simulink model "TAYCAN_MODEL"  (R2025b)
settings: Solver=ode23t  StartTime=0.0  StopTime=10000  RelTol=1e-3
values from neighbouring files (symbols this model uses):
  g = 9.81    [DRIVE_CYCLE_GEN.m]    (also in TAYCAN_PARAM_LOAD.m)
  L = 500    [TAYCAN_PARAM_LOAD.m]
  Max_brake_pressure_F_Bar = 200e5    (= 20000000)    [TAYCAN_PARAM_LOAD.m]
  Max_brake_pressure_R_Bar = 200e5    (= 20000000)    [TAYCAN_PARAM_LOAD.m]
  Max_torque_curve_F_Nm = Torque_x * Max_torque_curve_F_set    [Model_Sweeper.m]    (also in TAYCAN_PARAM_LOAD.m = [340;340;340;340;340;340;288.55;247.42;216.63;192.44;173.11;)
  Max_torque_curve_R_Nm = Torque_x * Max_torque_curve_R_set    [Model_Sweeper.m]    (also in TAYCAN_PARAM_LOAD.m = [900.00;900.00;900.00;900.00;900.00;900.00;900.00;898.90;785)
  Max_torque_generator_Nm = -350    [TAYCAN_PARAM_LOAD.m]
  Np = ceil(Ipack / Imax)    [Model_Sweeper.m]    (also in TAYCAN_PARAM_LOAD.m = 33)
  Ns = 198    [TAYCAN_PARAM_LOAD.m]
  regen_bias = 0.3    [TAYCAN_PARAM_LOAD.m]
  RPM_curve_RPM_F = (0:1000:RPM_max_RPM_F)'    [TAYCAN_PARAM_LOAD.m]
  RPM_curve_RPM_R = (0:1000:RPM_max_RPM_R)'    [TAYCAN_PARAM_LOAD.m]
  shift_down_v = shift_down_v_set(ids)    [Model_Sweeper.m]    (also in TAYCAN_PARAM_LOAD.m = 60)
  shift_up_v = shift_up_v_set(ids)    [Model_Sweeper.m]    (also in TAYCAN_PARAM_LOAD.m = 80)
  Tot_vehicle_mass_kg = Vehicle_mass_unladen_kg + Driver_mass_kg + batt_mass    [Model_Sweeper.m]    (also in TAYCAN_PARAM_LOAD.m = 2462.38)
  V_init = 4.2    [TAYCAN_PARAM_LOAD.m]
  VelDist = struct()    [DRIVE_CYCLE_GEN.m]    (also in VelocityVsDistance.mat = )
undefined symbols (not defined in the file or in its folder): Driver_Ki, Driver_Kp, Max_torque_motor_F__Nm, Max_torque_motor_R__Nm, Neg, Pos
libraries: fl_lib x23, nesl_utility x16, sdl_lib x15, batteryecm_lib x1, autolibshared x1
(part 2 of 2)

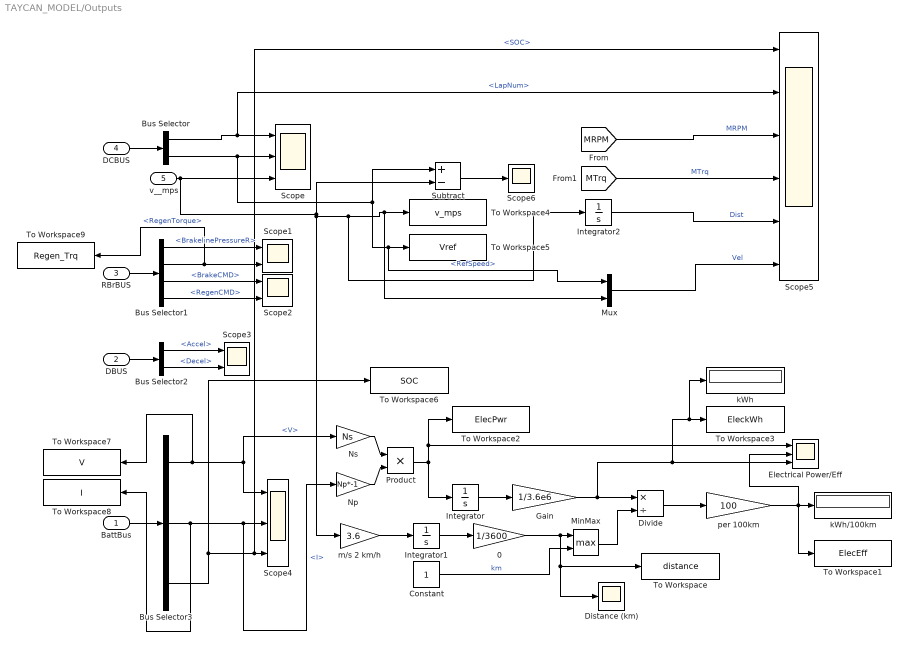
== system TAYCAN_MODEL/Outputs ==
  BattBus : Inport
  DBUS : Inport  Port=2
  RBrBUS : Inport  Port=3
  DCBUS : Inport  Port=4
  v__mps : Inport  Port=5
  0 : Gain  Gain=1/3600
  Bus Selector : BusSelector  OutputSignals=LapNum,RefSpeed
  Bus Selector1 : BusSelector  OutputSignals=BrakelinePressureR,RegenTorque,BrakeCMD,RegenCMD
  Bus Selector2 : BusSelector  OutputSignals=Info.Accel,Info.Decel
  Bus Selector3 : BusSelector  OutputSignals=V,I,SOC
  Constant : Constant
  Distance (km) : Scope
      settings: DataLoggingVariableName=ScopeData8
  Divide : Product  Inputs=*/
  Electrical Power/Eff : Scope  NumInputPorts=3
      settings: DataLoggingVariableName=ScopeData7
  Gain : Gain  Gain=1/3.6e6
  Integrator : Integrator
  Integrator1 : Integrator
  Integrator2 : Integrator
  MinMax : MinMax  Function=max  Inputs=2
  Mux : Mux  Inputs=2
  Np : Gain  Gain=Np*-1
  Ns : Gain  Gain=Ns
  Product : Product
  Scope : Scope  NumInputPorts=3
      settings: ActiveDisplayYMinimum=-0.24999999999999994  ActiveDisplayYMaximum=2.25
  Scope1 : Scope  NumInputPorts=2
      settings: ActiveDisplayYMinimum=-2.4999999999999995E+6  ActiveDisplayYMaximum=2.25E+7
  Scope2 : Scope  NumInputPorts=2
      settings: ActiveDisplayYMinimum=-0.087499999999999981  ActiveDisplayYMaximum=0.7875  DataLoggingVariableName=ScopeData2
  Scope3 : Scope  NumInputPorts=2
      settings: ActiveDisplayYMinimum=-0.12499999999999997  ActiveDisplayYMaximum=1.125  DataLoggingVariableName=ScopeData3
  Scope4 : Scope  NumInputPorts=3
      settings: ActiveDisplayYMinimum=1.4182763065735668  ActiveDisplayYMaximum=4.8626794045097581  DataLoggingVariableName=ScopeData4
  Scope5 : Scope  NumInputPorts=6
      settings: ActiveDisplayYMinimum=0.63060484486680279  ActiveDisplayYMaximum=0.81648445711282258  DataLoggingVariableName=ScopeData6
  Scope6 : Scope
      settings: ActiveDisplayYMinimum=-58.874697621468819  ActiveDisplayYMaximum=25.807756510642971  DataLoggingVariableName=ScopeData9
  Subtract : Sum  Inputs=+-
  To Workspace : ToWorkspace  VariableName=distance  SaveFormat=Timeseries  SampleTime=-1
  To Workspace1 : ToWorkspace  VariableName=ElecEff  SaveFormat=Timeseries  SampleTime=-1
  To Workspace2 : ToWorkspace  VariableName=ElecPwr  SaveFormat=Timeseries  SampleTime=-1
  To Workspace3 : ToWorkspace  VariableName=EleckWh  SaveFormat=Timeseries  SampleTime=-1
  To Workspace4 : ToWorkspace  VariableName=v_mps  SaveFormat=Timeseries  SampleTime=-1
  To Workspace5 : ToWorkspace  VariableName=Vref  SaveFormat=Timeseries  SampleTime=-1
  To Workspace6 : ToWorkspace  VariableName=SOC  SaveFormat=Timeseries  SampleTime=-1
  To Workspace7 : ToWorkspace  VariableName=V  SaveFormat=Timeseries  SampleTime=-1
  To Workspace8 : ToWorkspace  VariableName=I  SaveFormat=Timeseries  SampleTime=-1
  To Workspace9 : ToWorkspace  VariableName=Regen_Trq  SaveFormat=Timeseries  SampleTime=-1
  kWh : Display
  kWh/100km : Display
  m/s 2 km/h : Gain  Gain=3.6
  per 100km : Gain  Gain=100
  wires:
  DCBUS/1 -> Bus Selector/1
  RBrBUS/1 -> Bus Selector1/1
  DBUS/1 -> Bus Selector2/1
  BattBus/1 -> Bus Selector3/1
  Bus Selector/1 -> Scope5/2, Scope/1  "<LapNum>"
  Bus Selector1/1 -> Scope1/1  "<BrakelinePressureR>"
  Bus Selector1/2 -> To Workspace9/1, Scope1/2  "<RegenTorque>"
  Bus Selector1/4 -> Scope2/2  "<RegenCMD>"
  Bus Selector1/3 -> Scope2/1  "<BrakeCMD>"
  Bus Selector2/1 -> Scope3/1  "<Accel>"
  Bus Selector2/2 -> Scope3/2  "<Decel>"
  Bus Selector3/1 -> To Workspace7/1, Ns/1, Scope4/1  "<V>"
  Bus Selector3/2 -> To Workspace8/1, Scope4/2, Np/1  "<I>"
  Bus Selector/2 -> Mux/1, To Workspace5/1, Subtract/1, Scope/2  "<RefSpeed>"
  Product/1 -> Integrator/1, To Workspace2/1, Electrical Power/Eff/1
  Integrator/1 -> Gain/1
  Gain/1 -> Divide/1, kWh/1, To Workspace3/1, Electrical Power/Eff/3
  MinMax/1 -> Divide/2
  Constant/1 -> MinMax/2  "km"
  v__mps/1 -> Scope/3, Integrator2/1, Mux/2, To Workspace4/1, m/s 2 km/h/1, Subtract/2
  m/s 2 km/h/1 -> Integrator1/1
  Integrator1/1 -> 0/1
  0/1 -> Distance (km)/1, To Workspace/1, MinMax/1
  per 100km/1 -> To Workspace1/1, Electrical Power/Eff/2, kWh/100km/1
  Np/1 -> Product/2
  Ns/1 -> Product/1
  Subtract/1 -> Scope6/1
  Divide/1 -> per 100km/1
  [MRPM] -> Scope5/3  "MRPM"
  [MTrq] -> Scope5/4  "MTrq"
  Integrator2/1 -> Scope5/5  "Dist"
  Mux/1 -> Scope5/6  "Vel"
  Bus Selector3/3 -> To Workspace6/1, Scope5/1, Scope4/3  "<SOC>"

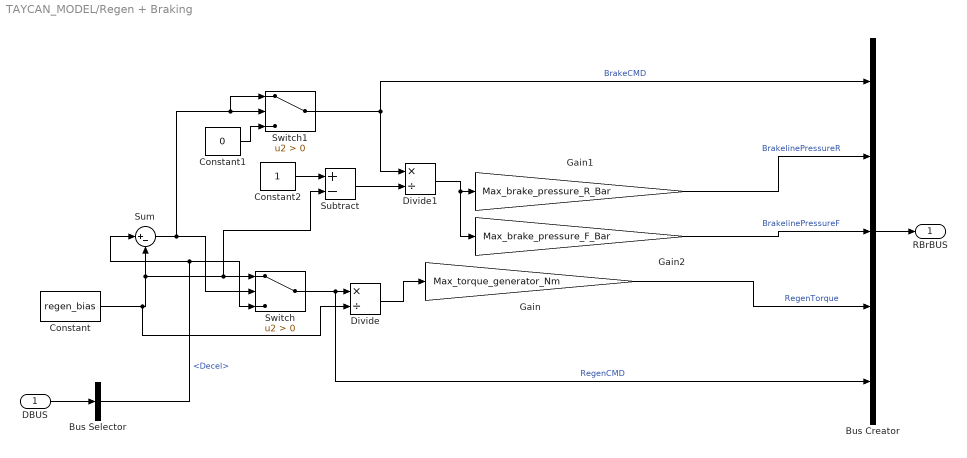
== system TAYCAN_MODEL/Regen + Braking ==
  DBUS : Inport
  Bus Creator : BusCreator  Inputs=5
  Bus Selector : BusSelector  OutputSignals=Info.Decel
  Constant : Constant  Value=regen_bias
  Constant1 : Constant  Value=0
  Constant2 : Constant
  Divide : Product  Inputs=*/
  Divide1 : Product  Inputs=*/
  Gain : Gain  Gain=Max_torque_generator_Nm
  Gain1 : Gain  Gain=Max_brake_pressure_R_Bar
  Gain2 : Gain  Gain=Max_brake_pressure_F_Bar
  Subtract : Sum  Inputs=+-
  Sum : Sum  Inputs=|+-
  Switch : Switch  Criteria=u2 > Threshold  SaturateOnIntegerOverflow=off  InputSameDT=off
  Switch1 : Switch  Criteria=u2 > Threshold  SaturateOnIntegerOverflow=off  InputSameDT=off
  RBrBUS : Outport
  wires:
  DBUS/1 -> Bus Selector/1
  Gain2/1 -> Bus Creator/3  "BrakelinePressureF"
  Gain/1 -> Bus Creator/4  "RegenTorque"
  Bus Creator/1 -> RBrBUS/1
  Gain1/1 -> Bus Creator/2  "BrakelinePressureR"
  Switch/1 -> Bus Creator/5, Divide/1  "RegenCMD"
  Switch1/1 -> Divide1/1, Bus Creator/1  "BrakeCMD"
  Constant2/1 -> Subtract/1
  Bus Selector/1 -> Sum/1, Switch/3  "<Decel>"
  Divide/1 -> Gain/1
  Sum/1 -> Switch1/1, Switch1/2, Switch/2
  Divide1/1 -> Gain1/1, Gain2/1
  Constant/1 -> Divide/2, Sum/2, Subtract/2, Switch/1
  Subtract/1 -> Divide1/2
  Constant1/1 -> Switch1/3

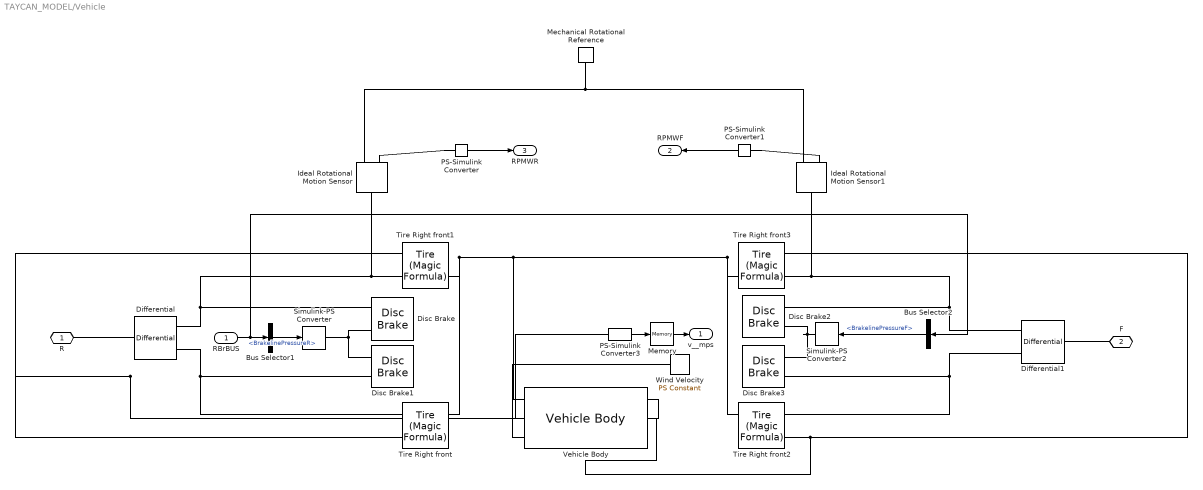
== system TAYCAN_MODEL/Vehicle ==
  RBrBUS : Inport
  Bus Selector1 : BusSelector  OutputSignals=BrakelinePressureR
  Bus Selector2 : BusSelector  OutputSignals=BrakelinePressureF
  Differential : sdl_lib/Gears/Differential  driveshaft_location=sdl.enum.differential_orientation.right  cd_ratio=Final_drive_ratio_R  friction_model=sdl.enum.gear_friction.none  efficiency=[.85, .92]  temperature_TLU=[280, 300, 320] K  efficiency_ss_TLU=[.95, .9, .85]  efficiency_cd_TLU=[.95, .9, .85]  pwr_thr=[.001, .001] W  mu_visc=[0, 0] N*m*s/rad  model_inertia=simscape.enum.onoff.off  sun_inertia=1e-10 kg*m^2  sun_radius=0.01 m  carrier_inertia=0.001 kg*m^2  planet_inertia=0.001 kg*m^2  planet_mass=1e-10 kg  thermal_mass=50 J/K  T_init=300 K
  Differential1 : sdl_lib/Gears/Differential  driveshaft_location=sdl.enum.differential_orientation.right  cd_ratio=Final_drive_ratio_F  friction_model=sdl.enum.gear_friction.none  efficiency=[.85, .92]  temperature_TLU=[280, 300, 320] K  efficiency_ss_TLU=[.95, .9, .85]  efficiency_cd_TLU=[.95, .9, .85]  pwr_thr=[.001, .001] W  mu_visc=[0, 0] N*m*s/rad  model_inertia=simscape.enum.onoff.off  sun_inertia=1e-10 kg*m^2  sun_radius=0.01 m  carrier_inertia=0.001 kg*m^2  planet_inertia=0.001 kg*m^2  planet_mass=1e-10 kg  thermal_mass=50 J/K  T_init=300 K
  Disc Brake : sdl_lib/Brakes & Detents/Rotational/Disc Brake  r_mean=Brake_pad_radius_R_m m  bore=Cylinder_bore_R_m m  n_pads=2  thermal_port=simscape.enum.thermaleffects.omit  mu_static=Static_Cf  mu_coulomb=Coulomb_Cf  temperature_TLU=[280, 300, 320] K  mu_static_TLU=[.9, .8, .7]  mu_coulomb_TLU=[.8, .7, .6]  brkwy_vel=Break_Fric_v_rads rad/s  visc_coef=Viscous_Cf N*m*s/rad  thermal_mass=50 kJ/K  temperature_specify=off  temperature_priority=High  temperature=300 K  temperature_nominal_specify=off  temperature_nominal_value=1  temperature_nominal_unit=K
  Disc Brake1 : sdl_lib/Brakes & Detents/Rotational/Disc Brake  r_mean=Brake_pad_radius_R_m m  bore=Cylinder_bore_R_m m  n_pads=2  thermal_port=simscape.enum.thermaleffects.omit  mu_static=Static_Cf  mu_coulomb=Coulomb_Cf  temperature_TLU=[280, 300, 320] K  mu_static_TLU=[.9, .8, .7]  mu_coulomb_TLU=[.8, .7, .6]  brkwy_vel=Break_Fric_v_rads rad/s  visc_coef=Viscous_Cf N*m*s/rad  thermal_mass=50 kJ/K  temperature_specify=off  temperature_priority=High  temperature=300 K  temperature_nominal_specify=off  temperature_nominal_value=1  temperature_nominal_unit=K
  Disc Brake2 : sdl_lib/Brakes & Detents/Rotational/Disc Brake  r_mean=Brake_pad_radius_F_m m  bore=Cylinder_bore_F_m m  n_pads=2  thermal_port=simscape.enum.thermaleffects.omit  mu_static=Static_Cf  mu_coulomb=Coulomb_Cf  temperature_TLU=[280, 300, 320] K  mu_static_TLU=[.9, .8, .7]  mu_coulomb_TLU=[.8, .7, .6]  brkwy_vel=Break_Fric_v_rads rad/s  visc_coef=Viscous_Cf N*m*s/rad  thermal_mass=50 kJ/K  temperature_specify=off  temperature_priority=High  temperature=300 K  temperature_nominal_specify=off  temperature_nominal_value=1  temperature_nominal_unit=K
  Disc Brake3 : sdl_lib/Brakes & Detents/Rotational/Disc Brake  r_mean=Brake_pad_radius_F_m m  bore=Cylinder_bore_F_m m  n_pads=2  thermal_port=simscape.enum.thermaleffects.omit  mu_static=Static_Cf  mu_coulomb=Coulomb_Cf  temperature_TLU=[280, 300, 320] K  mu_static_TLU=[.9, .8, .7]  mu_coulomb_TLU=[.8, .7, .6]  brkwy_vel=Break_Fric_v_rads rad/s  visc_coef=Viscous_Cf N*m*s/rad  thermal_mass=50 kJ/K  temperature_specify=off  temperature_priority=High  temperature=300 K  temperature_nominal_specify=off  temperature_nominal_value=1  temperature_nominal_unit=K
  Ideal Rotational Motion Sensor : fl_lib/Mechanical/Mechanical Sensors/Ideal Rotational Motion Sensor  reference=foundation.enum.MeasurementReference.difference  acceleration_port=false  velocity_port=true  position_port=false  wrap_angle=false  offset=0 rad
      settings: InternalSimscapePortConfiguration="{\"Bottom\":[],\"Left\":[{\"id\":\"R\",\"label\":\"R\",\"type\":\"foundation.mechanical.rotational.rotational\"}],\"Right\":[{\"id\":\"C\",\"label\":\"C\",\"type\":\"foundation.mechanical.rotational.rotational\"},{\"id\":\"W\",\"label\":\"W\",\"type\":\"output\"}],\"Top\":[]}"
  Ideal Rotational Motion Sensor1 : fl_lib/Mechanical/Mechanical Sensors/Ideal Rotational Motion Sensor  reference=foundation.enum.MeasurementReference.difference  acceleration_port=false  velocity_port=true  position_port=false  wrap_angle=false  offset=0 rad
      settings: InternalSimscapePortConfiguration="{\"Bottom\":[],\"Left\":[{\"id\":\"R\",\"label\":\"R\",\"type\":\"foundation.mechanical.rotational.rotational\"}],\"Right\":[{\"id\":\"C\",\"label\":\"C\",\"type\":\"foundation.mechanical.rotational.rotational\"},{\"id\":\"W\",\"label\":\"W\",\"type\":\"output\"}],\"Top\":[]}"
  Mechanical Rotational Reference : fl_lib/Mechanical/Rotational Elements/Mechanical Rotational Reference
  Memory : Memory  LinearizeMemory=on  LinearizeAsDelay=on
  PS-Simulink Converter : nesl_utility/PS-Simulink Converter  PhysicalDomain=network_engine_domain  SubClassName=ps_output  LeftPortType=input  RightPortType=output  PseudoPeriodic=off  Frequencies=[]  VectorFormat=inherit  Unit=rpm  AffineConversion=off
  PS-Simulink Converter1 : nesl_utility/PS-Simulink Converter  PhysicalDomain=network_engine_domain  SubClassName=ps_output  LeftPortType=input  RightPortType=output  PseudoPeriodic=off  Frequencies=[]  VectorFormat=inherit  Unit=rpm  AffineConversion=off
  PS-Simulink Converter3 : nesl_utility/PS-Simulink Converter  PhysicalDomain=network_engine_domain  SubClassName=ps_output  LeftPortType=input  RightPortType=output  PseudoPeriodic=off  Frequencies=[]  VectorFormat=1-D array  Unit=m/s  AffineConversion=off
  Simulink-PS Converter : nesl_utility/Simulink-PS Converter  PhysicalDomain=network_engine_domain  SubClassName=ps_input  LeftPortType=input  RightPortType=output  PseudoPeriodic=off  Frequencies=[]  NoiseDistribution=none  NoiseParameters=[]  Unit=Pa  AffineConversion=off  FilteringAndDerivatives=zero  SimscapeFilterOrder=1  InputFilterTimeConstant=.001  UdotUserProvided=0
  Simulink-PS Converter2 : nesl_utility/Simulink-PS Converter  PhysicalDomain=network_engine_domain  SubClassName=ps_input  LeftPortType=input  RightPortType=output  PseudoPeriodic=off  Frequencies=[]  NoiseDistribution=none  NoiseParameters=[]  Unit=Pa  AffineConversion=off  FilteringAndDerivatives=zero  SimscapeFilterOrder=1  InputFilterTimeConstant=.001  UdotUserProvided=0
  Tire Right front : sdl_lib/Tires & Vehicles/Tire (Magic Formula)  parameterization=sdl.enum.magic_tire_model.peak  F_z1=Vertical_load_pirelli_R_N N  F_x1=Longitudinal_load_pirelli_R_N N  kappa1=Peak_tyre_slip_pirelli_R  B_m=10  C_m=1.9  D_m=1  E_m=0.97  fz0=4e+3 N  p_Cx=1.685  p_Dx=[ 1.21 -0.037 ]  p_Ex=[ 0.344 0.095 -0.02 0 ]  p_Kx=[ 21.51 -0.163 0.245 ]  p_Hx=[ -0.002 0.002 ]  p_Vx=[ 0 0 ]  rolling_radius_model=sdl.enum.RollingRadiusParameterization.Constant  r_e=wheel_radius__m m  r_0=0.3 m  breff=8.39  dreff=0.26  freff=0.074  q_re0=0.99  q_v1=0.008  longvl=17 m/s  cz=5e5 N/m  model_resistance=true  resistance_model=1  coeff=Tyre_Crr_pirelli  p_tire=2.5e+5 Pa  alpha=-0.003  beta=0.97  coeff_a=0.008399999999999999  coeff_b=6.2e-4 s/m  coeff_c=1.6e-4 s^2/m^2  p_tire0=240e3 Pa  fz0_resistance=4000 N  vH0=16 m/s  q_Sy=[.0082, 0, .0014, .001, 0, 0, 1.08, -.5]  v_thr=0.001 m/s  enable_scaling_coefficients=false  lfzO=1  lcx=1  lmux=1  lex=1  lkx=1  lhx=1  lvx=1  lmy=1  model_compliance=sdl.enum.compliance.off  stiffness=1e+6 N/m  damping=1000 N/(m/s)  model_inertia=1  inertia=1e-2 kg*m^2  initial_velocity=0 rad/s  vxlow=0.1 m/s  v_tr_thr=0.1*(0.1) m/s  kpumin=-1e5  kpumax=1e8
  Tire Right front1 : sdl_lib/Tires & Vehicles/Tire (Magic Formula)  parameterization=sdl.enum.magic_tire_model.peak  F_z1=Vertical_load_pirelli_R_N N  F_x1=Longitudinal_load_pirelli_R_N N  kappa1=Peak_tyre_slip_pirelli_R  B_m=10  C_m=1.9  D_m=1  E_m=0.97  fz0=4e+3 N  p_Cx=1.685  p_Dx=[ 1.21 -0.037 ]  p_Ex=[ 0.344 0.095 -0.02 0 ]  p_Kx=[ 21.51 -0.163 0.245 ]  p_Hx=[ -0.002 0.002 ]  p_Vx=[ 0 0 ]  rolling_radius_model=sdl.enum.RollingRadiusParameterization.Constant  r_e=wheel_radius__m m  r_0=0.3 m  breff=8.39  dreff=0.26  freff=0.074  q_re0=0.99  q_v1=0.008  longvl=17 m/s  cz=5e5 N/m  model_resistance=true  resistance_model=1  coeff=Tyre_Crr_pirelli  p_tire=2.5e+5 Pa  alpha=-0.003  beta=0.97  coeff_a=0.008399999999999999  coeff_b=6.2e-4 s/m  coeff_c=1.6e-4 s^2/m^2  p_tire0=240e3 Pa  fz0_resistance=4000 N  vH0=16 m/s  q_Sy=[.0082, 0, .0014, .001, 0, 0, 1.08, -.5]  v_thr=0.001 m/s  enable_scaling_coefficients=false  lfzO=1  lcx=1  lmux=1  lex=1  lkx=1  lhx=1  lvx=1  lmy=1  model_compliance=sdl.enum.compliance.off  stiffness=1e+6 N/m  damping=1000 N/(m/s)  model_inertia=1  inertia=1e-2 kg*m^2  initial_velocity=0 rad/s  vxlow=0.1 m/s  v_tr_thr=0.1*(0.1) m/s  kpumin=-1e5  kpumax=1e8
  Tire Right front2 : sdl_lib/Tires & Vehicles/Tire (Magic Formula)  parameterization=sdl.enum.magic_tire_model.peak  F_z1=Vertical_load_pirelli_F_N N  F_x1=Longitudinal_load_pirelli_F_N N  kappa1=Peak_tyre_slip_pirelli_F  B_m=10  C_m=1.9  D_m=1  E_m=0.97  fz0=4e+3 N  p_Cx=1.685  p_Dx=[ 1.21 -0.037 ]  p_Ex=[ 0.344 0.095 -0.02 0 ]  p_Kx=[ 21.51 -0.163 0.245 ]  p_Hx=[ -0.002 0.002 ]  p_Vx=[ 0 0 ]  rolling_radius_model=sdl.enum.RollingRadiusParameterization.Constant  r_e=wheel_radius__m m  r_0=0.3 m  breff=8.39  dreff=0.26  freff=0.074  q_re0=0.99  q_v1=0.008  longvl=17 m/s  cz=5e5 N/m  model_resistance=true  resistance_model=1  coeff=Tyre_Crr_pirelli  p_tire=2.5e+5 Pa  alpha=-0.003  beta=0.97  coeff_a=0.008399999999999999  coeff_b=6.2e-4 s/m  coeff_c=1.6e-4 s^2/m^2  p_tire0=240e3 Pa  fz0_resistance=4000 N  vH0=16 m/s  q_Sy=[.0082, 0, .0014, .001, 0, 0, 1.08, -.5]  v_thr=0.001 m/s  enable_scaling_coefficients=false  lfzO=1  lcx=1  lmux=1  lex=1  lkx=1  lhx=1  lvx=1  lmy=1  model_compliance=sdl.enum.compliance.off  stiffness=1e+6 N/m  damping=1000 N/(m/s)  model_inertia=1  inertia=1e-2 kg*m^2  initial_velocity=0 rad/s  vxlow=0.1 m/s  v_tr_thr=0.1*(0.1) m/s  kpumin=-1e5  kpumax=1e8
  Tire Right front3 : sdl_lib/Tires & Vehicles/Tire (Magic Formula)  parameterization=sdl.enum.magic_tire_model.peak  F_z1=Vertical_load_pirelli_F_N N  F_x1=Longitudinal_load_pirelli_F_N N  kappa1=Peak_tyre_slip_pirelli_F  B_m=10  C_m=1.9  D_m=1  E_m=0.97  fz0=4e+3 N  p_Cx=1.685  p_Dx=[ 1.21 -0.037 ]  p_Ex=[ 0.344 0.095 -0.02 0 ]  p_Kx=[ 21.51 -0.163 0.245 ]  p_Hx=[ -0.002 0.002 ]  p_Vx=[ 0 0 ]  rolling_radius_model=sdl.enum.RollingRadiusParameterization.Constant  r_e=wheel_radius__m m  r_0=0.3 m  breff=8.39  dreff=0.26  freff=0.074  q_re0=0.99  q_v1=0.008  longvl=17 m/s  cz=5e5 N/m  model_resistance=true  resistance_model=1  coeff=Tyre_Crr_pirelli  p_tire=2.5e+5 Pa  alpha=-0.003  beta=0.97  coeff_a=0.008399999999999999  coeff_b=6.2e-4 s/m  coeff_c=1.6e-4 s^2/m^2  p_tire0=240e3 Pa  fz0_resistance=4000 N  vH0=16 m/s  q_Sy=[.0082, 0, .0014, .001, 0, 0, 1.08, -.5]  v_thr=0.001 m/s  enable_scaling_coefficients=false  lfzO=1  lcx=1  lmux=1  lex=1  lkx=1  lhx=1  lvx=1  lmy=1  model_compliance=sdl.enum.compliance.off  stiffness=1e+6 N/m  damping=1000 N/(m/s)  model_inertia=1  inertia=1e-2 kg*m^2  initial_velocity=0 rad/s  vxlow=0.1 m/s  v_tr_thr=0.1*(0.1) m/s  kpumin=-1e5  kpumax=1e8
  Vehicle Body : sdl_lib/Tires & Vehicles/Vehicle Body  mass=Tot_vehicle_mass_kg kg  n_w=Axle_wheel_no  x_f=D_CoG_F_m m  x_r=D_CoG_R_m m  y_c=H_CoG_m m  mass_var=simscape.enum.onoff.off  g=9.81 m/s^2  liftoff_warning=0  area=vehicle_frontal_area__m2 m^2  Cd_var=false  Cd=Cd  rho=rho kg/m^3  model_pitch=false  inertia=4000 kg*m^2  suspension_model=1  k_f=1e4 N/m  b_f=1e4 N/(m/s)  k_r=1e4 N/m  b_r=1e4 N/(m/s)  k_f_TLU=[-2000, -1000, 0, 1000, 2000] N  x_f_TLU=[-.4, -.2, 0, .2, .4] m  b_f_TLU=[-200, -100, 0, 100, 200] N  v_f_TLU=[-4, -2, 0, 2, 4] m/s  k_r_TLU=[-2000, -1000, 0, 1000, 2000] N  x_r_TLU=[-.4, -.2, 0, .2, .4] m  b_r_TLU=[-200, -100, 0, 100, 200] N  v_r_TLU=[-4, -2, 0, 2, 4] m/s  interp_method=simscape.enum.interpolation.linear  extrap_method=simscape.enum.extrapolation.linear  model_hardstop=0  upper_bound_f=.25 m  lower_bound_f=-.25 m  stop_k_f=1e6 N/m  stop_b_f=150 N/(m/s)  upper_bound_r=.25 m  lower_bound_r=-.25 m  stop_k_r=1e6 N/m  stop_b_r=150 N/(m/s)  initial_pitch=0 rad  initial_pitch_rate=0 rad/s  v_specify=on  v_priority=High  v=0 m/s  v_nominal_specify=off  v_nominal_value=1  v_nominal_unit=m/s
      settings: InternalSimscapePortConfiguration="{\"Bottom\":[{\"id\":\"NR\",\"label\":\"NR\",\"type\":\"output\"},{\"id\":\"NF\",\"label\":\"NF\",\"type\":\"output\"},{\"id\":\"beta\",\"label\":\"beta\",\"type\":\"input\"}],\"Left\":[{\"id\":\"H\",\"label\":\"H\",\"type\":\"foundation.mechanical.translational.translational\"}],\"Right\":[],\"Top\":[{\"id\":\"V\",\"label\":\"V\",\"type\":\"output\"},{\"id\":\"wind\",\"label\":\"W\",\"type\":\"input\"}]}"
  Wind Velocity : fl_lib/Physical Signals/Sources/PS Constant  constant=0
  R : PMIOPort  Side=Left
  F : PMIOPort  Port=2  Side=Left
  v__mps : Outport  VectorParamsAs1DForOutWhenUnconnected=off
  RPMWF : Outport  Port=2
  RPMWR : Outport  Port=3
  wires:
  RBrBUS/1 -> Bus Selector2/1, Bus Selector1/1
  Bus Selector1/1 -> Simulink-PS Converter/1  "<BrakelinePressureR>"
  PS-Simulink Converter3/1 -> Memory/1
  Memory/1 -> v__mps/1
  Bus Selector2/1 -> Simulink-PS Converter2/1  "<BrakelinePressureF>"
  PS-Simulink Converter/1 -> RPMWR/1
  PS-Simulink Converter1/1 -> RPMWF/1
  connections:
  Vehicle Body/RConn1 -- Tire Right front/LConn1 -- Tire Right front1/LConn1
  Disc Brake1/LConn2 -- Tire Right front/LConn2 -- Differential/RConn1
  Disc Brake/LConn2 -- Tire Right front1/LConn2 -- Ideal Rotational Motion Sensor/LConn1 -- Differential/RConn2
  Vehicle Body/RConn2 -- Tire Right front3/LConn1 -- Tire Right front2/LConn1
  R/RConn1 -- Differential/LConn1
  PS-Simulink Converter3/LConn1 -- Vehicle Body/LConn2
  Wind Velocity/RConn1 -- Vehicle Body/LConn3
  Vehicle Body/LConn1 -- Tire Right front/RConn2 -- Tire Right front1/RConn2 -- Tire Right front3/RConn2 -- Tire Right front2/RConn2
  Differential1/RConn1 -- Tire Right front3/LConn2 -- Ideal Rotational Motion Sensor1/LConn1 -- Disc Brake2/LConn2
  Differential1/RConn2 -- Tire Right front2/LConn2 -- Disc Brake3/LConn2
  F/RConn1 -- Differential1/LConn1
  Simulink-PS Converter/RConn1 -- Disc Brake1/LConn1 -- Disc Brake/LConn1
  Simulink-PS Converter2/RConn1 -- Disc Brake2/LConn1 -- Disc Brake3/LConn1
  Mechanical Rotational Reference/LConn1 -- Ideal Rotational Motion Sensor/RConn1 -- Ideal Rotational Motion Sensor1/RConn1
  PS-Simulink Converter/LConn1 -- Ideal Rotational Motion Sensor/RConn2
  PS-Simulink Converter1/LConn1 -- Ideal Rotational Motion Sensor1/RConn2

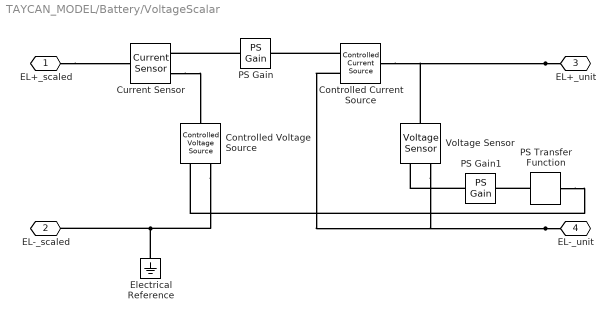
== system TAYCAN_MODEL/Battery/VoltageScalar ==
  Controlled Current Source : fl_lib/Electrical/Electrical Sources/Controlled Current Source
  Controlled Voltage Source : fl_lib/Electrical/Electrical Sources/Controlled Voltage Source
  Current Sensor : fl_lib/Electrical/Electrical Sensors/Current Sensor
  Electrical Reference : fl_lib/Electrical/Electrical Elements/Electrical Reference
  PS Gain : fl_lib/Physical Signals/Functions/PS Gain  gain=1/n_para
  PS Gain1 : fl_lib/Physical Signals/Functions/PS Gain  gain=n_ser
  PS Transfer Function : fl_lib/Physical Signals/Linear Operators/PS Transfer Function  transfer_function_type=foundation.enum.transfer_function_type.lag  T=t_filt s  T1=2 s  T2=1 s  reset_method=foundation.enum.IntegratorResetSpec.None  initial_condition_spec=foundation.enum.IntegratorICSpec.Internal  y0=V_init*n_ser V
      settings: InternalSimscapePortConfiguration="{\"Bottom\":[],\"Left\":[{\"id\":\"U\",\"label\":\"\",\"type\":\"input\"}],\"Right\":[{\"id\":\"Y\",\"label\":\"\",\"type\":\"output\"}],\"Top\":[]}"
  Voltage Sensor : fl_lib/Electrical/Electrical Sensors/Voltage Sensor
  EL+_scaled : PMIOPort  Side=Left
  EL-_scaled : PMIOPort  Port=2  Side=Left
  EL+_unit : PMIOPort  Port=3  Side=Right
  EL-_unit : PMIOPort  Port=4  Side=Right
  connections:
  EL+_scaled/RConn1 -- Current Sensor/LConn1
  Current Sensor/RConn2 -- Controlled Voltage Source/LConn1
  Controlled Voltage Source/RConn2 -- Electrical Reference/LConn1 -- EL-_scaled/RConn1
  PS Gain/LConn1 -- Current Sensor/RConn1
  Controlled Current Source/RConn1 -- PS Gain/RConn1
  EL+_unit/RConn1 -- Controlled Current Source/LConn1 -- Voltage Sensor/LConn1
  EL-_unit/RConn1 -- Controlled Current Source/RConn2 -- Voltage Sensor/RConn2
  PS Gain1/LConn1 -- Voltage Sensor/RConn1
  PS Transfer Function/LConn1 -- PS Gain1/RConn1
  PS Transfer Function/RConn1 -- Controlled Voltage Source/RConn1

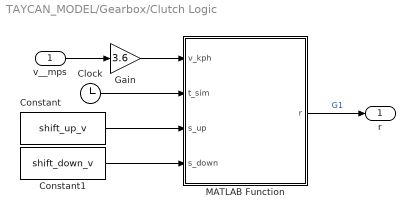
== system TAYCAN_MODEL/Gearbox/Clutch Logic ==
  v__mps : Inport
  Clock : Clock
  Constant : Constant  Value=shift_up_v
  Constant1 : Constant  Value=shift_down_v
  Gain : Gain  Gain=3.6
  MATLAB Function : MATLAB Function  TreatAsAtomicUnit=on
  r : Outport
  wires:
  v__mps/1 -> Gain/1
  Gain/1 -> MATLAB Function/1(v_kph)
  Clock/1 -> MATLAB Function/2(t_sim)
  Constant/1 -> MATLAB Function/3(s_up)
  Constant1/1 -> MATLAB Function/4(s_down)
  MATLAB Function/1(r) -> r/1  "G1"

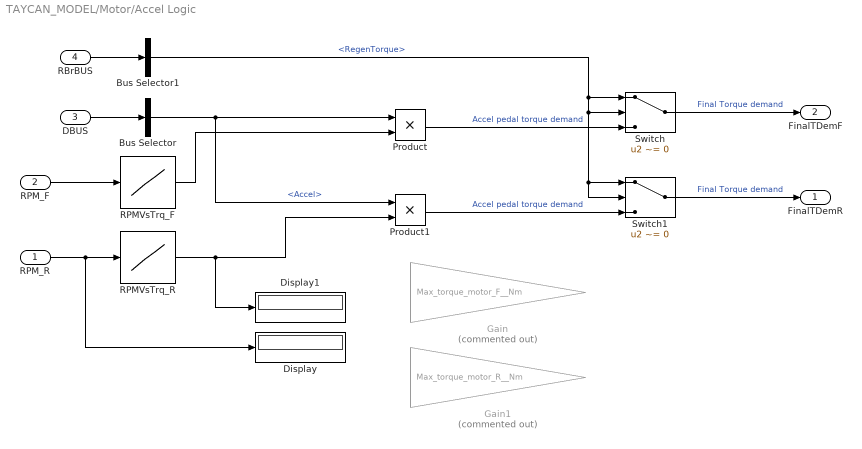
== system TAYCAN_MODEL/Motor/Accel Logic ==
  RPM_R : Inport
  RPM_F : Inport  Port=2
  DBUS : Inport  Port=3
  RBrBUS : Inport  Port=4
  Bus Selector : BusSelector  OutputSignals=Info.Accel
  Bus Selector1 : BusSelector  OutputSignals=RegenTorque
  Display : Display
  Display1 : Display
  Gain : Gain  Commented=on  Gain=Max_torque_motor_F__Nm
  Gain1 : Gain  Commented=on  Gain=Max_torque_motor_R__Nm
  Product : Product
  Product1 : Product
  RPMVsTrq_F : Lookup_n-D  NumberOfTableDimensions=1  BreakpointsForDimension1=RPM_curve_RPM_F  Table=Max_torque_curve_F_Nm  ExtrapMethod=Clip  InternalRulePriority=Speed  RndMeth=Simplest
  RPMVsTrq_R : Lookup_n-D  NumberOfTableDimensions=1  BreakpointsForDimension1=RPM_curve_RPM_R  Table=Max_torque_curve_R_Nm  ExtrapMethod=Clip  InternalRulePriority=Speed  RndMeth=Simplest
  Switch : Switch  Criteria=u2 ~= 0  SaturateOnIntegerOverflow=off  InputSameDT=off
  Switch1 : Switch  Criteria=u2 ~= 0  SaturateOnIntegerOverflow=off  InputSameDT=off
  FinalTDemR : Outport
  FinalTDemF : Outport  Port=2
  wires:
  Product/1 -> Switch/3  "Accel pedal torque demand"
  DBUS/1 -> Bus Selector/1
  Bus Selector/1 -> Product1/1, Product/1  "<Accel>"
  RBrBUS/1 -> Bus Selector1/1
  Bus Selector1/1 -> Switch/2, Switch1/2, Switch1/1, Switch/1  "<RegenTorque>"
  Switch/1 -> FinalTDemF/1  "Final Torque demand"
  Product1/1 -> Switch1/3  "Accel pedal torque demand"
  Switch1/1 -> FinalTDemR/1  "Final Torque demand"
  RPM_R/1 -> RPMVsTrq_R/1, Display/1
  RPM_F/1 -> RPMVsTrq_F/1
  RPMVsTrq_F/1 -> Product/2
  RPMVsTrq_R/1 -> Display1/1, Product1/2

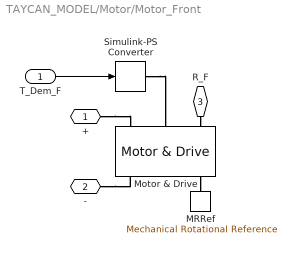
== system TAYCAN_MODEL/Motor/Motor_Front ==
  T_Dem_F : Inport
  MRRef : fl_lib/Mechanical/Rotational Elements/Mechanical Rotational Reference
  Motor & Drive : sdl_lib/Engines & Motors/Motor & Drive  torque_max=Max_torque_motor_F_Nm N*m  power_max=Max_power_motor_F_W W  Tc=Torque_control_T s  eff=Motor_eff_F  w_eff=RPM_measure_eff_F_RPM rpm  T_eff=Torque_measure_eff_F_Nm N*m  thermal_port=simscape.enum.thermaleffects.omit  thermal_mass=100 J/K  temperature_specify=off  temperature_priority=High  temperature=300 K  temperature_nominal_specify=off  temperature_nominal_value=1  temperature_nominal_unit=K
      settings: InternalSimscapePortConfiguration="{\"Bottom\":[],\"Left\":[{\"id\":\"Vp\",\"label\":\"+\",\"type\":\"foundation.electrical.electrical\"},{\"id\":\"Tr\",\"label\":\"Tr\",\"type\":\"input\"},{\"id\":\"R\",\"label\":\"R\",\"type\":\"foundation.mechanical.rotational.rotational\"}],\"Right\":[{\"id\":\"Vm\",\"label\":\"-\",\"type\":\"foundation.electrical.electrical\"},{\"id\":\"Omega\",\"label\":\"w\",\"type\":\"output\"},{\"id\":\"C\",\"label\":\"C\",\"type\":\"foundation.mechanical.rotational.rotational\"}],\"Top\":[]}"
  Simulink-PS Converter : nesl_utility/Simulink-PS Converter  PhysicalDomain=network_engine_domain  SubClassName=ps_input  LeftPortType=input  RightPortType=output  PseudoPeriodic=off  Frequencies=[]  NoiseDistribution=none  NoiseParameters=[]  Unit=N*m  AffineConversion=off  FilteringAndDerivatives=zero  SimscapeFilterOrder=1  InputFilterTimeConstant=.001  UdotUserProvided=0
  + : PMIOPort  Side=Left
  - : PMIOPort  Port=2  Side=Left
  R_F : PMIOPort  Port=3  Side=Right
  wires:
  T_Dem_F/1 -> Simulink-PS Converter/1
  connections:
  Motor & Drive/RConn3 -- MRRef/LConn1
  R_F/RConn1 -- Motor & Drive/LConn3
  +/RConn1 -- Motor & Drive/LConn1
  Simulink-PS Converter/RConn1 -- Motor & Drive/LConn2
  -/RConn1 -- Motor & Drive/RConn1

== system TAYCAN_MODEL/Motor/Motor_Rear ==
  T_Dem_R : Inport
  MRRef : fl_lib/Mechanical/Rotational Elements/Mechanical Rotational Reference
  Motor & Drive : sdl_lib/Engines & Motors/Motor & Drive  torque_max=Max_torque_motor_R_Nm N*m  power_max=Max_power_motor_R_W W  Tc=Torque_control_T s  eff=Motor_eff_R  w_eff=RPM_measure_eff_R_RPM rpm  T_eff=Torque_measure_eff_R_Nm N*m  thermal_port=simscape.enum.thermaleffects.omit  thermal_mass=100 J/K  temperature_specify=off  temperature_priority=High  temperature=300 K  temperature_nominal_specify=off  temperature_nominal_value=1  temperature_nominal_unit=K
      settings: InternalSimscapePortConfiguration="{\"Bottom\":[],\"Left\":[{\"id\":\"Vp\",\"label\":\"+\",\"type\":\"foundation.electrical.electrical\"},{\"id\":\"Tr\",\"label\":\"Tr\",\"type\":\"input\"},{\"id\":\"R\",\"label\":\"R\",\"type\":\"foundation.mechanical.rotational.rotational\"}],\"Right\":[{\"id\":\"Vm\",\"label\":\"-\",\"type\":\"foundation.electrical.electrical\"},{\"id\":\"Omega\",\"label\":\"w\",\"type\":\"output\"},{\"id\":\"C\",\"label\":\"C\",\"type\":\"foundation.mechanical.rotational.rotational\"}],\"Top\":[]}"
  Simulink-PS Converter : nesl_utility/Simulink-PS Converter  PhysicalDomain=network_engine_domain  SubClassName=ps_input  LeftPortType=input  RightPortType=output  PseudoPeriodic=off  Frequencies=[]  NoiseDistribution=none  NoiseParameters=[]  Unit=N*m  AffineConversion=off  FilteringAndDerivatives=zero  SimscapeFilterOrder=1  InputFilterTimeConstant=.001  UdotUserProvided=0
  + : PMIOPort  Side=Left
  - : PMIOPort  Port=2  Side=Left
  R_R : PMIOPort  Port=3  Side=Right
  wires:
  T_Dem_R/1 -> Simulink-PS Converter/1
  connections:
  Motor & Drive/RConn3 -- MRRef/LConn1
  Simulink-PS Converter/RConn1 -- Motor & Drive/LConn2
  +/RConn1 -- Motor & Drive/LConn1
  -/RConn1 -- Motor & Drive/RConn1
  R_R/RConn1 -- Motor & Drive/LConn3

== matlab function TAYCAN_MODEL/Gearbox/Clutch Logic/MATLAB Function ==
  settings: updateMethod=DISCRETE
  data: v_kph input; r output; t_sim input; s_up input; s_down input
% function [G1, G2] = shiftLogic(v_kph, t_sim,s_up, s_down)
% % Speed-based 2-speed shift logic with hysteresis + break-before-make delay
% % Adds a startup hold so Simscape IC solver always sees a valid torque path
% 
% % ---- tunables ----
% v_up    = s_up;     % km/h (1 -> 2)
% v_down  = s_down;     % km/h (2 -> 1)
% shiftDelay = 0.10; % seconds break-before-make
% Ts = 0.01;         % controller sample time
% tHold = 0.05;      % seconds: force G1 engaged at startup to help IC solve
% 
% % ---- persistent state ----
% persistent gear targetGear shifting tshift
% if isempty(gear)
%     gear = 1;
%     targetGear = 1;
%     shifting = false;
%     tshift = 0;
% end
% 
% % ---- HARD STARTUP CONDITION (important for Simscape IC solve) ----
% % Simulink/Simscape may call this multiple times at t=0 while initializing.
% % So we force a consistent engaged gear for the whole tHold window.
% if t_sim < tHold
%     gear = 1;
%     targetGear = 1;
%     shifting = false;
%     tshift = 0;
%     G1 = 1;
%     G2 = 0;
%     return;
% end
% 
% % ---- decide target gear (hysteresis) ----
% if ~shifting
%     if gear == 1 && v_kph > v_up
%         targetGear = 2;
%         shifting = true;
%         tshift = 0;
%     elseif gear == 2 && v_kph < v_down
%         targetGear = 1;
%         shifting = true;
%         tshift = 0;
%     end
% end
% 
% % ---- break-before-make sequence ----
% if shifting
%     tshift = tshift + Ts;
% 
%     if tshift < shiftDelay
%         % both open (break)
%         G1 = 0;
%         G2 = 0;
%     else
%         % engage target (make)
%         gear = targetGear;
%         shifting = false;
% 
%         G1 = double(gear == 1);
%         G2 = double(gear == 2);
%     end
% else
%     % steady state
%     G1 = double(gear == 1);
%     G2 = double(gear == 2);
% end
% 

function r = shiftLogicRatio(v_kph, t_sim, s_up, s_down)
% Outputs a single ratio r for a Variable Ratio Transmission block
% Gear 1: r = 15
% Gear 2: r = 8
% Includes hysteresis + smooth ratio transition to help Simscape convergence

% ---- ratios ----
r1 = 15;   % 1st gear ratio
r2 = 8;    % 2nd gear ratio

% ---- shift thresholds ----
v_up   = s_up;    % km/h, 1 -> 2
v_down = s_down;  % km/h, 2 -> 1

% ---- timing ----
tHold     = 0.05; % s, force gear 1 at startup (IC help)
shiftTime = 0.10; % s, blend time for ratio change (solver-friendly)

% ---- persistent state ----
persistent gear shifting tStart rStart rTarget
if isempty(gear)
    gear = 1;
    shifting = false;
    tStart = 0;
    rStart = r1;
    rTarget = r1;
end

% ---- hard startup hold ----
if t_sim < tHold
    gear = 1;
    shifting = false;
    r = r1;
    rStart = r1;
    rTarget = r1;
    return;
end

% ---- decide shift target (hysteresis) ----
if ~shifting
    if gear == 1 && v_kph > v_up
        gear = 2;                % update gear state immediately
        shifting = true;
        tStart = t_sim;
        rStart = r1;
        rTarget = r2;
    elseif gear == 2 && v_kph < v_down
        gear = 1;
        shifting = true;
        tStart = t_sim;
        rStart = r2;
        rTarget = r1;
    end
end

% ---- smooth transition of ratio ----
if shifting
    alpha = (t_sim - tStart) / shiftTime;
    if alpha >= 1
        r = rTarget;
        shifting = false;
    else
        % linear blend (you can swap for smootherstep if you want)
        r = rStart + alpha * (rTarget - rStart);
    end
else
    r = (gear == 1) * r1 + (gear == 2) * r2;
end
